simulink model "project3"  (R2022a)
settings: Solver=VariableStepAuto  StartTime=0.0  StopTime=10.0  RelTol=1e-3
values from neighbouring files (symbols this model uses):
  b = 0.73.88.169.153    [project3_run.m]
  F = 1    [project3_run.m]
  k = 20    [project3_run.m]
  M = 1    [project3_run.m]
settings Model: Creator=DDYD  LastModifiedBy=DDYD

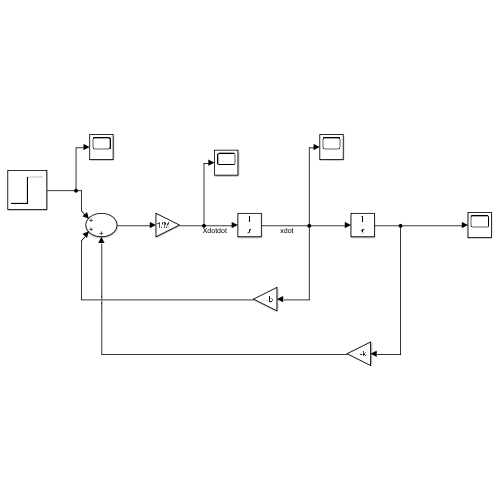
[thumbnail: Simulink's stored preview of the top-level diagram]
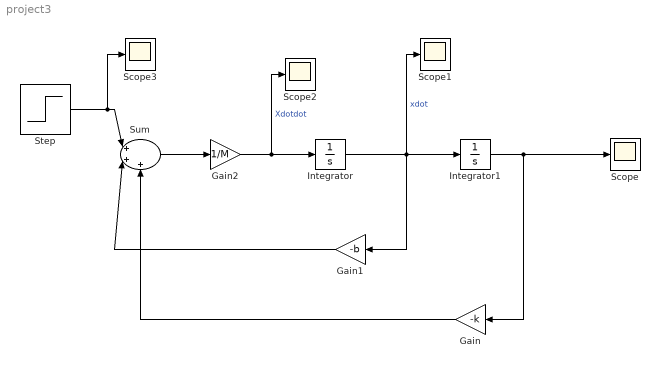
== system project3 ==
  Gain : Gain  Gain=-k
  Gain1 : Gain  Gain=-b
  Gain2 : Gain  Gain=1/M
  Integrator : Integrator
  Integrator1 : Integrator
  Scope{,1..3} (4 alike) : Scope
  Step : Step  After=F  SampleTime=0
  Sum : Sum  Inputs=|+++
  wires:
  Gain2/1 -> Scope2/1, Integrator/1  "Xdotdot"
  Integrator/1 -> Scope1/1, Gain1/1, Integrator1/1  "xdot"
  Integrator1/1 -> Scope/1, Gain/1
  Step/1 -> Scope3/1, Sum/1
  Gain1/1 -> Sum/2
  Gain/1 -> Sum/3
  Sum/1 -> Gain2/1
